simulink model "robot_control"  (R2022b)
settings: Solver=FixedStepAuto  StartTime=0.0  StopTime=30  RelTol=1e-3
undefined symbols (not defined in the file or in its folder): ODR
libraries: raspberrypiBasiclib x6, raspberrypiIMUsensorslib x2, simulink x1
settings Model: Creator=sjohnson  LastModifiedBy=sjohnson
settings SolverCC: PositivePriorityOrder=on
settings OptimizationCC: EnhancedBackFolding=on  PassReuseOutputArgsAs=Individual arguments  ZeroExternalMemoryAtStartup=off  ZeroInternalMemoryAtStartup=off  MaxStackSize=64  OptimizeBlockOrder=speed  DifferentSizesBufferReuse=on  OptimizationCustomize=off  EfficientTunableParamExpr=on
settings DebuggingCC: ParameterTunabilityLossMsg=error
settings HardwareCC: ProdBitPerPointer=32  ProdBitPerSizeT=32  ProdBitPerPtrDiffT=32  ProdLargestAtomicInteger=Long  ProdLargestAtomicFloat=Double  ProdWordSize=32  ProdLongLongMode=on  ProdHWDeviceType=ARM Compatible->ARM Cortex  UseEmbeddedCoderFeatures=off  UseSimulinkCoderFeatures=off
settings ModelReferenceCC: EnableParallelModelReferenceBuilds=on
settings RTWCC: Description=Embedded Coder  SystemTargetFile=ert.tlc  HardwareBoard=Raspberry Pi  TLCOptions="-aInlineSetEventsForThisBaseRateFcn=TLC_FALSE -aSuppressMultiTaskScheduler=TLC_FALSE  -aRateBasedStepFcn=0"  TemplateMakefile=ert_default_tmf  Toolchain=GNU GCC Embedded Linux  BuildConfiguration=Faster Runs
settings CodeAppCC: ForceParamTrailComments=on  IgnoreCustomStorageClasses=off  OperatorAnnotations=on  SimulinkDataObjDesc=on  SFDataObjDesc=on  MangleLength=10  InsertBlockDesc=on
settings ERTTargetCC: SupportNonInlinedSFcns=on  SupportVariableSizeSignals=on  ExtModeTransport=2  ExtModeStaticAlloc=on  ExtModeMexFile=ext_xcp  ExtModeIntrfLevel=Level2 - Open

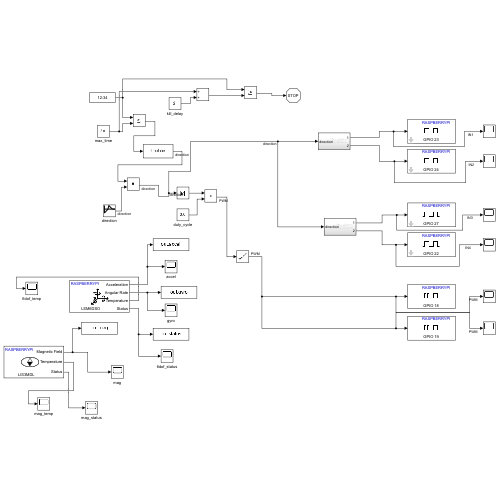
[thumbnail: Simulink's stored preview of the top-level diagram]
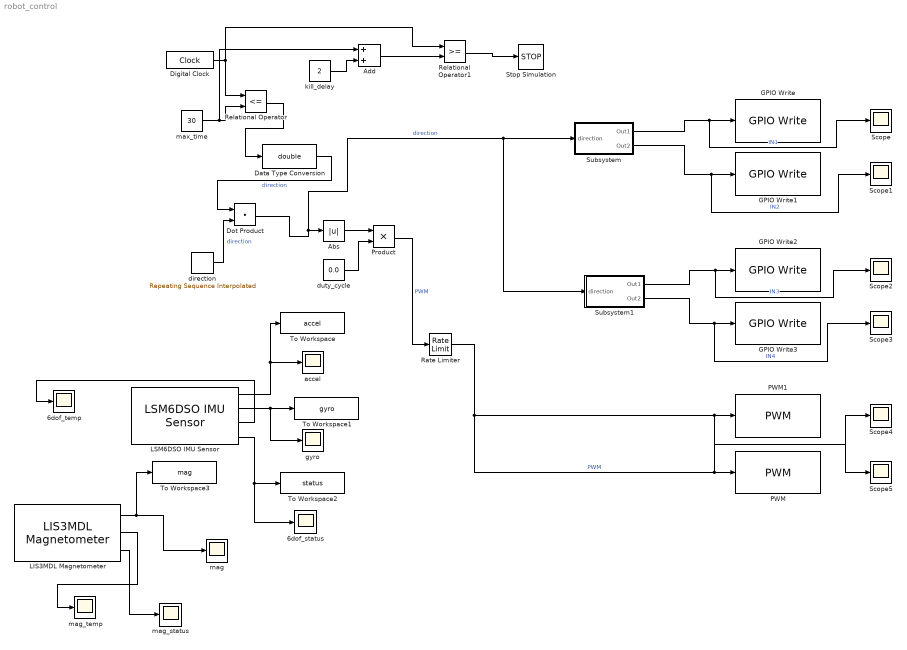
== system robot_control ==
  6dof_status : Scope
  6dof_temp : Scope
  Abs : Abs  SaturateOnIntegerOverflow=off
  Add : Sum
  Data Type Conversion : DataTypeConversion  OutDataTypeStr=double  SaturateOnIntegerOverflow=off  RndMeth=Floor  LockScale=on
  Digital Clock : DigitalClock  SampleTime=.1
  Dot Product : DotProduct  OutDataTypeStr=Inherit: Inherit via internal rule
  GPIO Write : raspberrypiBasiclib/GPIO Write  board=Pi 4 Model B  gpio=23  direction=Output  blockPlatform=Raspberry Pi
  GPIO Write1 : raspberrypiBasiclib/GPIO Write  board=Pi 4 Model B  gpio=24  direction=Output  blockPlatform=Raspberry Pi
  GPIO Write2 : raspberrypiBasiclib/GPIO Write  board=Pi 4 Model B  gpio=27  direction=Output  blockPlatform=Raspberry Pi
  GPIO Write3 : raspberrypiBasiclib/GPIO Write  board=Pi 4 Model B  gpio=22  direction=Output  blockPlatform=Raspberry Pi
  LIS3MDL Magnetometer : raspberrypiIMUsensorslib/LIS3MDL Magnetometer  I2CModule=1  I2CAddress=0x1E  IsActiveMagnetometer=on  IsActiveTemperature=on  IsStatus=on  SampleTime=-1  MagnetometerRange=+/- 400 uT  MagnetometerODR=155 Hz
  LSM6DSO IMU Sensor : raspberrypiIMUsensorslib/LSM6DSO IMU Sensor  I2CModule=1  I2CAddress=0x6B  IsActiveAcceleration=on  IsActiveAngularRate=on  IsActiveTemperature=on  IsActiveStatus=on  IsActiveTimeStamp=off  SampleTime=-1  QueueSizeFactor=3  AccelerometerRange=+/- 2g  AccelerometerODR=104 Hz  AccelSelectCompositeFilter=No filter  AccelLPF2BW=ODR/4  AccelHPFBW=ODR/4  GyroscopeRange=125 dps  GyroscopeODR=104 Hz  EnableGyroHPF=off  GyroHPFBW=0.016 Hz  EnableGyroLPF=off  GyroLPFBWMode=0
  PWM : raspberrypiBasiclib/PWM  board=Pi 4 Model B  Pin_=19  Frequency=50  blockPlatform=Raspberry Pi
  PWM1 : raspberrypiBasiclib/PWM  board=Pi 4 Model B  Pin_=18  Frequency=50  blockPlatform=Raspberry Pi
  Product : Product
  Rate Limiter : RateLimiter  RisingSlewLimit=2  FallingSlewLimit=-2  SampleTimeMode=inherited
  Relational Operator : RelationalOperator  Operator=<=  OutDataTypeStr=boolean  RndMeth=Simplest  InputSameDT=off
  Relational Operator1 : RelationalOperator  OutDataTypeStr=boolean  RndMeth=Simplest  InputSameDT=off
  Scope{,1..5} (6 alike) : Scope
  Stop Simulation : Stop
  Subsystem : Subsystem
  Subsystem1 : Subsystem
  To Workspace : ToWorkspace  VariableName=accel  SaveFormat=Structure With Time  SampleTime=-1
  To Workspace1 : ToWorkspace  VariableName=gyro  SaveFormat=Structure With Time  SampleTime=-1
  To Workspace2 : ToWorkspace  VariableName=status  SaveFormat=Structure With Time  SampleTime=-1
  To Workspace3 : ToWorkspace  VariableName=mag  SaveFormat=Structure With Time  SampleTime=-1
  accel : Scope
  direction : simulink/Sources/Repeating Sequence Interpolated  OutValues=[-1 0 1 0 0].'  TimeValues=[0 1.0 1.25 2.25 3].'  LookUpMeth=Use Input Below  tsamp=0.01  OutMin=[]  OutMax=[]  OutDataTypeStr=double  OutputDataTypeScalingMode=double  OutDataType=fixdt(0,8)  OutScaling=2^-10
  duty_cycle : Constant  Value=0.0
  gyro : Scope
  kill_delay : Constant  Value=2
  mag : Scope
  mag_status : Scope
  mag_temp : Scope
  max_time : Constant  Value=30
  wires:
  Dot Product/1 -> Subsystem1/1(direction), Subsystem/1(direction), Abs/1  "direction"
  duty_cycle/1 -> Product/2
  Abs/1 -> Product/1
  Rate Limiter/1 -> Scope5/1, PWM/1, Scope4/1, PWM1/1  "PWM"
  Subsystem/1(Out1) -> Scope/1, GPIO Write/1  "IN1"
  Subsystem/2(Out2) -> Scope1/1, GPIO Write1/1  "IN2"
  Subsystem1/1(Out1) -> Scope2/1, GPIO Write2/1  "IN3"
  Subsystem1/2(Out2) -> Scope3/1, GPIO Write3/1  "IN4"
  Digital Clock/1 -> Relational Operator1/1, Relational Operator/1
  max_time/1 -> Add/1, Relational Operator/2
  Data Type Conversion/1 -> Dot Product/1  "direction"
  direction/1 -> Dot Product/2  "direction"
  Relational Operator/1 -> Data Type Conversion/1
  kill_delay/1 -> Add/2
  Add/1 -> Relational Operator1/2
  Relational Operator1/1 -> Stop Simulation/1
  Product/1 -> Rate Limiter/1  "PWM"
  LSM6DSO IMU Sensor/1 -> accel/1, To Workspace/1
  LSM6DSO IMU Sensor/2 -> gyro/1, To Workspace1/1
  LSM6DSO IMU Sensor/4 -> To Workspace2/1, 6dof_status/1
  LIS3MDL Magnetometer/1 -> To Workspace3/1, mag/1
  LSM6DSO IMU Sensor/3 -> 6dof_temp/1
  LIS3MDL Magnetometer/2 -> mag_temp/1
  LIS3MDL Magnetometer/3 -> mag_status/1

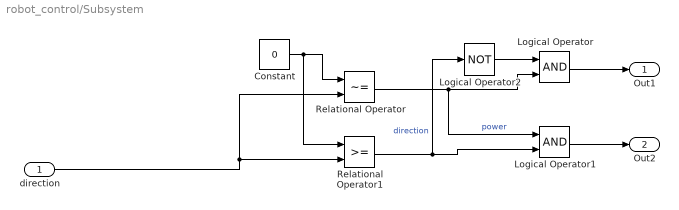
== system robot_control/Subsystem ==
  direction : Inport
  Constant : Constant  Value=0
  Logical Operator : Logic  AllPortsSameDT=off  OutDataTypeStr=boolean
  Logical Operator1 : Logic  AllPortsSameDT=off  OutDataTypeStr=boolean
  Logical Operator2 : Logic  Operator=NOT  Inputs=1  AllPortsSameDT=off  OutDataTypeStr=boolean
  Relational Operator : RelationalOperator  Operator=~=  OutDataTypeStr=boolean  RndMeth=Simplest  InputSameDT=off
  Relational Operator1 : RelationalOperator  OutDataTypeStr=boolean  RndMeth=Simplest  InputSameDT=off
  Out1 : Outport
  Out2 : Outport  Port=2
  wires:
  Logical Operator/1 -> Out1/1
  Relational Operator1/1 -> Logical Operator2/1, Logical Operator1/2  "direction"
  Logical Operator1/1 -> Out2/1
  Logical Operator2/1 -> Logical Operator/1
  direction/1 -> Relational Operator/2, Relational Operator1/2
  Constant/1 -> Relational Operator1/1, Relational Operator/1
  Relational Operator/1 -> Logical Operator1/1, Logical Operator/2  "power"

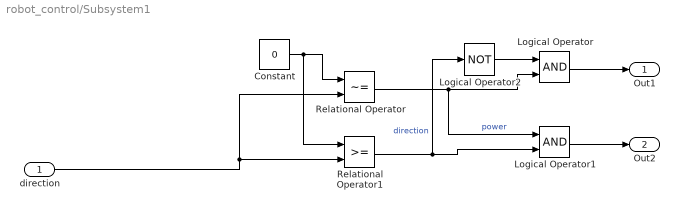
== system robot_control/Subsystem1 ==
  direction : Inport
  Constant : Constant  Value=0
  Logical Operator : Logic  AllPortsSameDT=off  OutDataTypeStr=boolean
  Logical Operator1 : Logic  AllPortsSameDT=off  OutDataTypeStr=boolean
  Logical Operator2 : Logic  Operator=NOT  Inputs=1  AllPortsSameDT=off  OutDataTypeStr=boolean
  Relational Operator : RelationalOperator  Operator=~=  OutDataTypeStr=boolean  RndMeth=Simplest  InputSameDT=off
  Relational Operator1 : RelationalOperator  OutDataTypeStr=boolean  RndMeth=Simplest  InputSameDT=off
  Out1 : Outport
  Out2 : Outport  Port=2
  wires:
  Logical Operator/1 -> Out1/1
  Relational Operator1/1 -> Logical Operator2/1, Logical Operator1/2  "direction"
  Logical Operator1/1 -> Out2/1
  Logical Operator2/1 -> Logical Operator/1
  direction/1 -> Relational Operator/2, Relational Operator1/2
  Constant/1 -> Relational Operator1/1, Relational Operator/1
  Relational Operator/1 -> Logical Operator1/1, Logical Operator/2  "power"
